simulink model "HT07CombinedPowertrainThermalModel"  (R2022b)
settings: Solver=VariableStepAuto  StartTime=0.0  StopTime=timeEnd  RelTol=1e-4
values from neighbouring files (symbols this model uses):
  Tamb = 26    [HT07CombinedPowertrainThermalSetupExperimental.m]
undefined symbols (not defined in the file or in its folder): AH, convectionArea, DiscIntNeverNeededParam, radiator, SOC0, startTempC, tabResis
libraries: fl_lib x161, nesl_utility x40, SimscapeFluids_lib x16, ee_lib x2
(part 1 of 5)
settings Model: Creator=erc  LastModifiedBy=David
settings SolverCC: MaxConsecutiveMinStep=10
settings DebuggingCC: UnconnectedInputMsg=warning  UnconnectedOutputMsg=warning  UnconnectedLineMsg=warning
settings ModelReferenceCC: EnableRefExpFcnMdlSchedulingChecks=on
settings RTWCC: DLArmComputeVersion=19.05

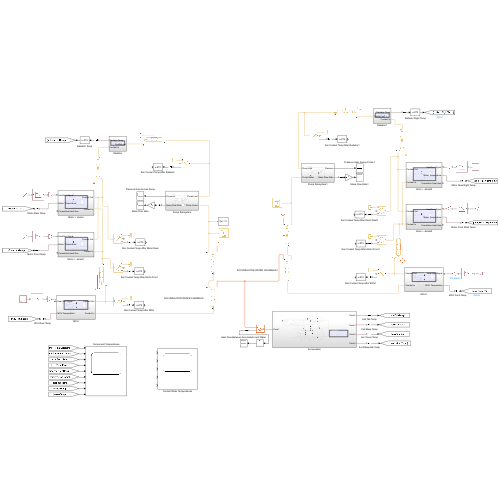
[thumbnail: Simulink's stored preview of the top-level diagram]
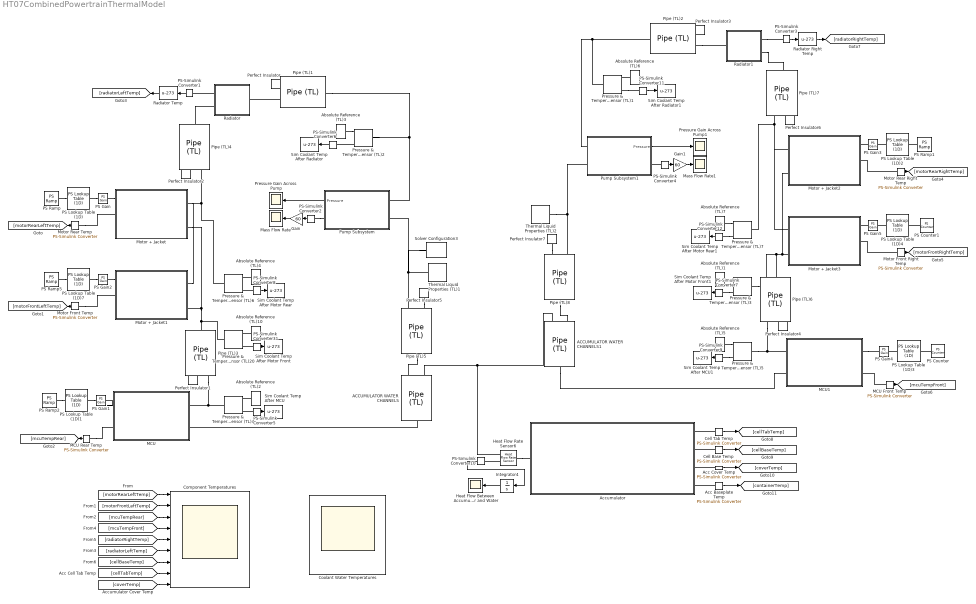
== system HT07CombinedPowertrainThermalModel ==
  ACCUMULATOR WATER CHANNELS : SimscapeFluids_lib/Thermal Liquid/Pipes & Fittings/Pipe (TL)  dynamic_compressibility=simscape.enum.onoff.off  inertia=simscape.enum.onoff.off  num_segments=1  pipe_length=accChannelLength m  area=accChannelFlowArea m^2  wall_spec=fluids.thermal_liquid.pipes_fittings.enum.wall_spec.rigid  Dh=accChannelHydraulicDiameter m  wall_compliance=1.2e-6 m/MPa  wall_time_constant=0.01 s  elevation_spec=foundation.enum.constant_variable.constant  elevation_gain=0 m  g=9.81 m/s^2  pressure_loss_spec=fluids.thermal_liquid.pipes_fittings.enum.PressureLossSpec.Haaland  local_pressure_loss_spec=fluids.thermal_liquid.pipes_fittings.enum.LocalLossSpec.AggregateLength  length_add=0 m  loss_coefficient=0.1  roughness=accChannelAbsoluteRoughness m  Re_friction_TLU=[400, 1000, 1500, 3000, 4000, 6000, 10000, 20000, 40000, 60000, 100000, 100000000]  friction_factor_TLU=[.264, .112, .071, .0417, .0387, .0268, .025, .0232, .0226, .022, .0214, .0214]  shape_factor=64  Re_lam=2000  Re_tur=4000  mdot_nominal=7 kg/min  p_diff_nominal=0.6 bar  mdot_threshold=1e-6 kg/s  heat_transfer_spec=fluids.thermal_liquid.pipes_fittings.enum.HeatTransferSpec.DittusBoelter  mdot_nominal_heat=[.1, 1] kg/s  T_in_nominal=[293.15, 293.15] K  T_out_nominal=[300, 300] K  p_in_nominal_heat=[.101325, .101325] MPa  T_wall_nominal=[303.15, 303.15] K  a_coeff=dittusBoelterAadjAccChannel  b_Re_power=0.8  c_Pr_power=0.4  Nu_lam=3.66  Re_Colburn_TLU=[100, 150, 1000]  Colburn_factor_TLU=[.019, .013, .002]  Re_Nu_TLU=[100, 150, 1000]  Pr_Nu_TLU=[1, 10]  Nu_TLU=[3.72, 4.21; 3.75, 4.44; 4.21, 7.15]  T0_vec=Tamb degC  p0_vec=0.101325 MPa  mdot0=0.1 kg/s
  ACCUMULATOR WATER CHANNELS1 : SimscapeFluids_lib/Thermal Liquid/Pipes & Fittings/Pipe (TL)  dynamic_compressibility=simscape.enum.onoff.off  inertia=simscape.enum.onoff.off  num_segments=1  pipe_length=accChannelLength m  area=accChannelFlowArea m^2  wall_spec=fluids.thermal_liquid.pipes_fittings.enum.wall_spec.rigid  Dh=accChannelHydraulicDiameter m  wall_compliance=1.2e-6 m/MPa  wall_time_constant=0.01 s  elevation_spec=foundation.enum.constant_variable.constant  elevation_gain=0 m  g=9.81 m/s^2  pressure_loss_spec=fluids.thermal_liquid.pipes_fittings.enum.PressureLossSpec.Haaland  local_pressure_loss_spec=fluids.thermal_liquid.pipes_fittings.enum.LocalLossSpec.AggregateLength  length_add=0 m  loss_coefficient=0.1  roughness=accChannelAbsoluteRoughness m  Re_friction_TLU=[400, 1000, 1500, 3000, 4000, 6000, 10000, 20000, 40000, 60000, 100000, 100000000]  friction_factor_TLU=[.264, .112, .071, .0417, .0387, .0268, .025, .0232, .0226, .022, .0214, .0214]  shape_factor=64  Re_lam=2000  Re_tur=4000  mdot_nominal=7 kg/min  p_diff_nominal=0.6 bar  mdot_threshold=1e-6 kg/s  heat_transfer_spec=fluids.thermal_liquid.pipes_fittings.enum.HeatTransferSpec.DittusBoelter  mdot_nominal_heat=[.1, 1] kg/s  T_in_nominal=[293.15, 293.15] K  T_out_nominal=[300, 300] K  p_in_nominal_heat=[.101325, .101325] MPa  T_wall_nominal=[303.15, 303.15] K  a_coeff=dittusBoelterAadjAccChannel  b_Re_power=0.8  c_Pr_power=0.4  Nu_lam=3.66  Re_Colburn_TLU=[100, 150, 1000]  Colburn_factor_TLU=[.019, .013, .002]  Re_Nu_TLU=[100, 150, 1000]  Pr_Nu_TLU=[1, 10]  Nu_TLU=[3.72, 4.21; 3.75, 4.44; 4.21, 7.15]  T0_vec=Tamb degC  p0_vec=0.101325 MPa  mdot0=0.1 kg/s
  Absolute Reference (TL){1..7,10} (8 alike) : fl_lib/Thermal Liquid/Elements/Absolute Reference (TL)
  Acc Baseplate Temp : nesl_utility/PS-Simulink Converter  PhysicalDomain=network_engine_domain  SubClassName=ps_output  LeftPortType=input  RightPortType=output  PseudoPeriodic=off  Frequencies=[]  VectorFormat=inherit  Unit=inherit  AffineConversion=off
  Acc Cover Temp : nesl_utility/PS-Simulink Converter  PhysicalDomain=network_engine_domain  SubClassName=ps_output  LeftPortType=input  RightPortType=output  PseudoPeriodic=off  Frequencies=[]  VectorFormat=inherit  Unit=inherit  AffineConversion=off
  Accumulator : Subsystem
  Cell Base Temp : nesl_utility/PS-Simulink Converter  PhysicalDomain=network_engine_domain  SubClassName=ps_output  LeftPortType=input  RightPortType=output  PseudoPeriodic=off  Frequencies=[]  VectorFormat=inherit  Unit=inherit  AffineConversion=off
  Cell Tab Temp : nesl_utility/PS-Simulink Converter  PhysicalDomain=network_engine_domain  SubClassName=ps_output  LeftPortType=input  RightPortType=output  PseudoPeriodic=off  Frequencies=[]  VectorFormat=inherit  Unit=inherit  AffineConversion=off
  Component Temperatures : Scope  NumInputPorts=9
  Coolant Water Temperatures : Scope  NumInputPorts=5
  Gain : Gain  Gain=60
  Gain1 : Gain  Gain=60
  Heat Flow Between Accumulator and Water : Scope
  Heat Flow Rate Sensor6 : fl_lib/Thermal/Thermal Sensors/Heat Flow Rate Sensor
  Integrator4 : Integrator
  MCU : Subsystem
  MCU Front Temp : nesl_utility/PS-Simulink Converter  PhysicalDomain=network_engine_domain  SubClassName=ps_output  LeftPortType=input  RightPortType=output  PseudoPeriodic=off  Frequencies=[]  VectorFormat=inherit  Unit=inherit  AffineConversion=off
  MCU Rear Temp : nesl_utility/PS-Simulink Converter  PhysicalDomain=network_engine_domain  SubClassName=ps_output  LeftPortType=input  RightPortType=output  PseudoPeriodic=off  Frequencies=[]  VectorFormat=inherit  Unit=inherit  AffineConversion=off
  MCU1 : Subsystem
  Mass Flow Rate : Scope
  Mass Flow Rate1 : Scope
  Motor + Jacket : Subsystem
  Motor + Jacket1 : Subsystem
  Motor + Jacket2 : Subsystem
  Motor + Jacket3 : Subsystem
  Motor Front Right Temp : nesl_utility/PS-Simulink Converter  PhysicalDomain=network_engine_domain  SubClassName=ps_output  LeftPortType=input  RightPortType=output  PseudoPeriodic=off  Frequencies=[]  VectorFormat=inherit  Unit=inherit  AffineConversion=off
  Motor Front Temp : nesl_utility/PS-Simulink Converter  PhysicalDomain=network_engine_domain  SubClassName=ps_output  LeftPortType=input  RightPortType=output  PseudoPeriodic=off  Frequencies=[]  VectorFormat=inherit  Unit=inherit  AffineConversion=off
  Motor Rear Right Temp : nesl_utility/PS-Simulink Converter  PhysicalDomain=network_engine_domain  SubClassName=ps_output  LeftPortType=input  RightPortType=output  PseudoPeriodic=off  Frequencies=[]  VectorFormat=inherit  Unit=inherit  AffineConversion=off
  Motor Rear Temp : nesl_utility/PS-Simulink Converter  PhysicalDomain=network_engine_domain  SubClassName=ps_output  LeftPortType=input  RightPortType=output  PseudoPeriodic=off  Frequencies=[]  VectorFormat=inherit  Unit=inherit  AffineConversion=off
  PS Counter : fl_lib/Physical Signals/Sources/PS Counter  sample_time=1 s  init_val=0  reset_val=0  max_val=intmax
      settings: InternalSimscapePortConfiguration="{\"Bottom\":[],\"Left\":[],\"Right\":[{\"id\":\"Y\",\"label\":\"Y\",\"type\":\"output\"}],\"Top\":[]}"
  PS Counter1 : fl_lib/Physical Signals/Sources/PS Counter  sample_time=1 s  init_val=0  reset_val=0  max_val=intmax
      settings: InternalSimscapePortConfiguration="{\"Bottom\":[],\"Left\":[],\"Right\":[{\"id\":\"Y\",\"label\":\"Y\",\"type\":\"output\"}],\"Top\":[]}"
  PS Gain{,2..3,5} (4 alike) : fl_lib/Physical Signals/Functions/PS Gain  gain=1
  PS Gain1 : fl_lib/Physical Signals/Functions/PS Gain  gain=2
  PS Gain4 : fl_lib/Physical Signals/Functions/PS Gain  gain=2
  PS Lookup Table (1D) : fl_lib/Physical Signals/Lookup Tables/PS Lookup Table (1D)  x=time  f=motorRearHeatGen J/s  interp_method=simscape.enum.interpolation.linear  extrap_method=simscape.enum.extrapolation.nearest
  PS Lookup Table (1D)1 : fl_lib/Physical Signals/Lookup Tables/PS Lookup Table (1D)  x=time  f=mcuHeatGen J/s  interp_method=simscape.enum.interpolation.linear  extrap_method=simscape.enum.extrapolation.nearest
  PS Lookup Table (1D)2 : fl_lib/Physical Signals/Lookup Tables/PS Lookup Table (1D)  x=time  f=motorRearHeatGen J/s  interp_method=simscape.enum.interpolation.linear  extrap_method=simscape.enum.extrapolation.nearest
  PS Lookup Table (1D)3 : fl_lib/Physical Signals/Lookup Tables/PS Lookup Table (1D)  x=time  f=mcuHeatGen J/s  interp_method=simscape.enum.interpolation.linear  extrap_method=simscape.enum.extrapolation.nearest
  PS Lookup Table (1D)4 : fl_lib/Physical Signals/Lookup Tables/PS Lookup Table (1D)  x=time  f=motorFrontHeatGen J/s  interp_method=simscape.enum.interpolation.linear  extrap_method=simscape.enum.extrapolation.nearest
  PS Lookup Table (1D)7 : fl_lib/Physical Signals/Lookup Tables/PS Lookup Table (1D)  x=time  f=motorFrontHeatGen J/s  interp_method=simscape.enum.interpolation.linear  extrap_method=simscape.enum.extrapolation.nearest
  PS Ramp{,1..2,5} (4 alike) : fl_lib/Physical Signals/Sources/PS Ramp  slope=1 1/s  start_time=0 s  initial_output=0
  PS-Simulink Converter{1,3,5..9,11..12,31} (10 alike) : nesl_utility/PS-Simulink Converter  PhysicalDomain=network_engine_domain  SubClassName=ps_output  LeftPortType=input  RightPortType=output  PseudoPeriodic=off  Frequencies=[]  VectorFormat=inherit  Unit=inherit  AffineConversion=off
  PS-Simulink Converter10 : nesl_utility/PS-Simulink Converter  PhysicalDomain=network_engine_domain  SubClassName=ps_output  LeftPortType=input  RightPortType=output  PseudoPeriodic=off  Frequencies=[]  VectorFormat=1-D array  Unit=inherit  AffineConversion=off
  PS-Simulink Converter2 : nesl_utility/PS-Simulink Converter  PhysicalDomain=network_engine_domain  SubClassName=ps_output  LeftPortType=input  RightPortType=output  PseudoPeriodic=off  Frequencies=[]  VectorFormat=1-D array  Unit=inherit  AffineConversion=off
  PS-Simulink Converter4 : nesl_utility/PS-Simulink Converter  PhysicalDomain=network_engine_domain  SubClassName=ps_output  LeftPortType=input  RightPortType=output  PseudoPeriodic=off  Frequencies=[]  VectorFormat=1-D array  Unit=inherit  AffineConversion=off
  Perfect Insulator{,1..7} (8 alike) : fl_lib/Thermal/Thermal Elements/Perfect Insulator  T_specify=off  T_priority=None  T=0 K  T_nominal_specify=off  T_nominal_unit=K  T_nominal_value=1
  Pipe (TL)1 : fl_lib/Thermal Liquid/Elements/Pipe (TL)  length=tubeLengthRadiatorToPump m  area=A m^2  Dh=d m  length_add=0 m  roughness=tubeRoughness m  Re_lam=2000  Re_tur=4000  shape_factor=64  Nu_lam=3.66  dynamic_compressibility=simscape.enum.onoff.off  inertia=simscape.enum.onoff.off  p0=0.101325 MPa  T0=Tamb degC  mdot0=0 kg/s
  Pipe (TL)2 : fl_lib/Thermal Liquid/Elements/Pipe (TL)  length=tubeLengthRadiatorToPump m  area=A m^2  Dh=d m  length_add=0 m  roughness=tubeRoughness m  Re_lam=2000  Re_tur=4000  shape_factor=64  Nu_lam=3.66  dynamic_compressibility=simscape.enum.onoff.off  inertia=simscape.enum.onoff.off  p0=0.101325 MPa  T0=Tamb degC  mdot0=0 kg/s
  Pipe (TL)3 : fl_lib/Thermal Liquid/Elements/Pipe (TL)  length=tubeLengthMCUToMotor m  area=A m^2  Dh=d m  length_add=leqMCUToMotor m  roughness=tubeRoughness m  Re_lam=2000  Re_tur=4000  shape_factor=64  Nu_lam=3.66  dynamic_compressibility=simscape.enum.onoff.off  inertia=simscape.enum.onoff.off  p0=0.101325 MPa  T0=Tamb degC  mdot0=0 kg/s
  Pipe (TL)4 : fl_lib/Thermal Liquid/Elements/Pipe (TL)  length=tubeLengthMotorToRadiator m  area=A m^2  Dh=d m  length_add=leqMotorToRadiator m  roughness=tubeRoughness m  Re_lam=2000  Re_tur=4000  shape_factor=64  Nu_lam=3.66  dynamic_compressibility=simscape.enum.onoff.off  inertia=simscape.enum.onoff.off  p0=0.101325 MPa  T0=Tamb degC  mdot0=0 kg/s
  Pipe (TL)5 : fl_lib/Thermal Liquid/Elements/Pipe (TL)  length=tubeLengthPumpToMCU m  area=A m^2  Dh=d m  length_add=leqMCUToMotor m  roughness=tubeRoughness m  Re_lam=2000  Re_tur=4000  shape_factor=64  Nu_lam=3.66  dynamic_compressibility=simscape.enum.onoff.off  inertia=simscape.enum.onoff.off  p0=0.101325 MPa  T0=Tamb degC  mdot0=0 kg/s
  Pipe (TL)6 : fl_lib/Thermal Liquid/Elements/Pipe (TL)  length=tubeLengthMCUToMotor m  area=A m^2  Dh=d m  length_add=leqMCUToMotor m  roughness=tubeRoughness m  Re_lam=2000  Re_tur=4000  shape_factor=64  Nu_lam=3.66  dynamic_compressibility=simscape.enum.onoff.off  inertia=simscape.enum.onoff.off  p0=0.101325 MPa  T0=Tamb degC  mdot0=0 kg/s
  Pipe (TL)7 : fl_lib/Thermal Liquid/Elements/Pipe (TL)  length=tubeLengthMotorToRadiator m  area=A m^2  Dh=d m  length_add=leqMotorToRadiator m  roughness=tubeRoughness m  Re_lam=2000  Re_tur=4000  shape_factor=64  Nu_lam=3.66  dynamic_compressibility=simscape.enum.onoff.off  inertia=simscape.enum.onoff.off  p0=0.101325 MPa  T0=Tamb degC  mdot0=0 kg/s
  Pipe (TL)8 : fl_lib/Thermal Liquid/Elements/Pipe (TL)  length=tubeLengthPumpToMCU m  area=A m^2  Dh=d m  length_add=leqMCUToMotor m  roughness=tubeRoughness m  Re_lam=2000  Re_tur=4000  shape_factor=64  Nu_lam=3.66  dynamic_compressibility=simscape.enum.onoff.off  inertia=simscape.enum.onoff.off  p0=0.101325 MPa  T0=Tamb degC  mdot0=0 kg/s
  Pressure & Temperature Sensor (TL){1..7,20} (8 alike) : fl_lib/Thermal Liquid/Sensors/Pressure & Temperature Sensor (TL)
      settings: InternalSimscapePortConfiguration="{\"Bottom\":[],\"Left\":[{\"id\":\"A\",\"label\":\"A\",\"type\":\"foundation.thermal_liquid.thermal_liquid\"}],\"Right\":[{\"id\":\"B\",\"label\":\"B\",\"type\":\"foundation.thermal_liquid.thermal_liquid\"},{\"id\":\"P\",\"label\":\"P\",\"type\":\"output\"},{\"id\":\"T\",\"label\":\"T\",\"type\":\"output\"}],\"Top\":[]}"
  Pressure Gain Across Pump : Scope
  Pressure Gain Across Pump1 : Scope
  Pump Subsystem : Subsystem
  Pump Subsystem1 : Subsystem
  Radiator : Subsystem
  Radiator Right Temp : Bias  Bias=-273  SaturateOnIntegerOverflow=off
  Radiator Temp : Bias  Bias=-273  SaturateOnIntegerOverflow=off
  Radiator1 : Subsystem
  Sim Coolant Temp After MCU : Bias  Bias=-273  SaturateOnIntegerOverflow=off
  Sim Coolant Temp After MCU1 : Bias  Bias=-273  SaturateOnIntegerOverflow=off
  Sim Coolant Temp After Motor Front : Bias  Bias=-273  SaturateOnIntegerOverflow=off
  Sim Coolant Temp After Motor Front1 : Bias  Bias=-273  SaturateOnIntegerOverflow=off
  Sim Coolant Temp After Motor Rear : Bias  Bias=-273  SaturateOnIntegerOverflow=off
  Sim Coolant Temp After Motor Rear1 : Bias  Bias=-273  SaturateOnIntegerOverflow=off
  Sim Coolant Temp After Radiator : Bias  Bias=-273  SaturateOnIntegerOverflow=off
  Sim Coolant Temp After Radiator1 : Bias  Bias=-273  SaturateOnIntegerOverflow=off
  Solver Configuration3 : nesl_utility/Solver Configuration  PhysicalDomain=network_engine_domain  SubClassName=solver  LeftPortType=input  RightPortType=generic  Tones=[]  Harmonics=[]  SimulateNoise=off  Profile=off  UseLocalSampling=off  EnableSwitchedLinearOptims=on  FrequencyDomain=off  UseCCode=off  RelTol=0.001  AbsTol=1e-06  MinStep=1e-09  ToWorkspace=off  RevertToSquareIcSolve=off  NumHomotopyIterations=100  PhasorMode=off  PhasorModeNumHarmonics=1  ConsistencySolver=NEWTON_FTOL  IndexReductionMethod=DerivativeReplacement  DoDC=on  ResidualTolerance=1e-08  ConsistencyTolSource=GLOBAL  ConsistencyAbsTol=0.001  ConsistencyRelTol=0.001  ConsistencyTolFactor=0.001  UseLocalSolver=off  LocalSolverChoice=NE_BACKWARD_EULER_ADVANCER  ResolveIndetEquations=on  FunctionEvalNumThread=1  LocalSolverSampleTime=0.001  DoFixedCost=off  MaxNonlinIter=3  MaxModeIter=2  ComputeImpulses=off  ImpulseIterations=2  LinearAlgebra=auto  LinearAlgebraNumThread=0  EquationFormulation=NE_TIME_EF  DelaysMemoryBudget=1024  AutomaticFiltering=on  FilteringTimeConstant=0.001  PartitionStorageMethod=AS_NEEDED  PartitionMemoryBudget=1024  PartitionMethod=ROBUST
  Thermal Liquid Properties (TL)1 : SimscapeFluids_lib/Thermal Liquid/Utilities/Thermal Liquid Properties (TL)  fluid_list=fluids.thermal_liquid.utilities.enum.thermal_liquid_fluid_list.water  concentration_param_EG=fluids.thermal_liquid.utilities.enum.thermal_liquid_concentration.volume_fraction  concentration_param_PG=fluids.thermal_liquid.utilities.enum.thermal_liquid_concentration.volume_fraction  c_mass_SW=3.5e-3  c_mass_EG=0.1  c_mass_PG=0.1  c_mass_GL=0.1  c_vol_EG=0.1  c_vol_PG=0.1  beta_const_EG=2.1791 GPa  beta_const_PG=2.1791 GPa  beta_const_GL=2.1791 GPa  p_min_EG=0.01 MPa  p_min_PG=0.01 MPa  p_min_GL=0.01 MPa  p_max_EG=50 MPa  p_max_PG=50 MPa  p_max_GL=50 MPa  p_atm=0.101325 MPa
  Thermal Liquid Properties (TL)2 : SimscapeFluids_lib/Thermal Liquid/Utilities/Thermal Liquid Properties (TL)  fluid_list=fluids.thermal_liquid.utilities.enum.thermal_liquid_fluid_list.water  concentration_param_EG=fluids.thermal_liquid.utilities.enum.thermal_liquid_concentration.volume_fraction  concentration_param_PG=fluids.thermal_liquid.utilities.enum.thermal_liquid_concentration.volume_fraction  c_mass_SW=3.5e-3  c_mass_EG=0.1  c_mass_PG=0.1  c_mass_GL=0.1  c_vol_EG=0.1  c_vol_PG=0.1  beta_const_EG=2.1791 GPa  beta_const_PG=2.1791 GPa  beta_const_GL=2.1791 GPa  p_min_EG=0.01 MPa  p_min_PG=0.01 MPa  p_min_GL=0.01 MPa  p_max_EG=50 MPa  p_max_PG=50 MPa  p_max_GL=50 MPa  p_atm=0.101325 MPa
  wires:
  PS-Simulink Converter6/1 -> Sim Coolant Temp After Radiator/1
  PS-Simulink Converter5/1 -> Sim Coolant Temp After MCU/1
  PS-Simulink Converter8/1 -> Sim Coolant Temp After Motor Rear/1
  PS-Simulink Converter31/1 -> Sim Coolant Temp After Motor Front/1
  Integrator4/1 -> Heat Flow Between Accumulator and Water/1
  PS-Simulink Converter10/1 -> Integrator4/1
  Motor Rear Temp/1 -> [motorRearLeftTemp]
  [motorRearLeftTemp] -> Component Temperatures/1
  Motor Front Temp/1 -> [motorFrontLeftTemp]
  [motorFrontLeftTemp] -> Component Temperatures/2
  MCU Rear Temp/1 -> [mcuTempRear]
  [mcuTempRear] -> Component Temperatures/3
  Pump Subsystem/1(Pressure) -> Pressure Gain Across Pump/1
  PS-Simulink Converter1/1 -> Radiator Temp/1
  [radiatorLeftTemp] -> Component Temperatures/6
  PS-Simulink Converter2/1 -> Gain/1
  Gain/1 -> Mass Flow Rate/1
  Radiator Temp/1 -> [radiatorLeftTemp]
  Motor Rear Right Temp/1 -> [motorRearRightTemp]
  PS-Simulink Converter7/1 -> Sim Coolant Temp After Motor Front1/1
  Motor Front Right Temp/1 -> [motorFrontRightTemp]
  PS-Simulink Converter9/1 -> Sim Coolant Temp After MCU1/1
  Pump Subsystem1/1(Pressure) -> Pressure Gain Across Pump1/1
  PS-Simulink Converter12/1 -> Sim Coolant Temp After Motor Rear1/1
  Gain1/1 -> Mass Flow Rate1/1
  PS-Simulink Converter4/1 -> Gain1/1
  Radiator Right Temp/1 -> [radiatorRightTemp]
  PS-Simulink Converter11/1 -> Sim Coolant Temp After Radiator1/1
  PS-Simulink Converter3/1 -> Radiator Right Temp/1
  MCU Front Temp/1 -> [mcuTempFront]
  [mcuTempFront] -> Component Temperatures/4
  Cell Tab Temp/1 -> [cellTabTemp]
  Cell Base Temp/1 -> [cellBaseTemp]
  Acc Cover Temp/1 -> [coverTemp]
  Acc Baseplate Temp/1 -> [containerTemp]
  [radiatorRightTemp] -> Component Temperatures/5
  [cellBaseTemp] -> Component Temperatures/7
  [coverTemp] -> Component Temperatures/9
  [cellTabTemp] -> Component Temperatures/8
  connections:
  PS Lookup Table (1D)1/RConn1 -- PS Gain1/LConn1
  PS Ramp2/RConn1 -- PS Lookup Table (1D)1/LConn1
  Perfect Insulator/LConn1 -- Pipe (TL)1/LConn2
  Thermal Liquid Properties (TL)1/RConn1 -- Solver Configuration3/RConn1 -- Pump Subsystem/LConn2 -- Pipe (TL)5/LConn1
  Absolute Reference (TL)3/LConn1 -- Pressure & Temperature Sensor (TL)2/RConn1
  Pressure & Temperature Sensor (TL)2/RConn3 -- PS-Simulink Converter6/LConn1
  Perfect Insulator1/LConn1 -- Pipe (TL)3/LConn2
  Pipe (TL)4/LConn2 -- Perfect Insulator2/LConn1
  Perfect Insulator5/LConn1 -- Pipe (TL)5/LConn2
  Pressure & Temperature Sensor (TL)6/LConn1 -- Motor + Jacket1/LConn1 -- Motor + Jacket/LConn1 -- Pipe (TL)4/LConn1
  ACCUMULATOR WATER CHANNELS/RConn1 -- MCU/RConn2
  Pipe (TL)3/LConn1 -- MCU/RConn1 -- Pressure & Temperature Sensor (TL)4/LConn1
  Absolute Reference (TL)2/LConn1 -- Pressure & Temperature Sensor (TL)4/RConn1
  PS-Simulink Converter5/LConn1 -- Pressure & Temperature Sensor (TL)4/RConn3
  Absolute Reference (TL)4/LConn1 -- Pressure & Temperature Sensor (TL)6/RConn1
  PS-Simulink Converter8/LConn1 -- Pressure & Temperature Sensor (TL)6/RConn3
  PS Lookup Table (1D)/RConn1 -- PS Gain/LConn1
  PS Ramp/RConn1 -- PS Lookup Table (1D)/LConn1
  PS Lookup Table (1D)7/RConn1 -- PS Gain2/LConn1
  PS Ramp5/RConn1 -- PS Lookup Table (1D)7/LConn1
  PS-Simulink Converter31/LConn1 -- Pressure & Temperature Sensor (TL)20/RConn3
  Absolute Reference (TL)10/LConn1 -- Pressure & Temperature Sensor (TL)20/RConn1
  Pipe (TL)5/RConn1 -- ACCUMULATOR WATER CHANNELS/LConn1
  Heat Flow Rate Sensor6/RConn1 -- PS-Simulink Converter10/LConn1
  ACCUMULATOR WATER CHANNELS/LConn2 -- ACCUMULATOR WATER CHANNELS1/LConn2 -- Heat Flow Rate Sensor6/RConn2
  Pressure & Temperature Sensor (TL)20/LConn1 -- Motor + Jacket/LConn2 -- Motor + Jacket1/LConn2 -- Pipe (TL)3/RConn1
  Pipe (TL)1/LConn1 -- Radiator/LConn1
  Radiator/RConn2 -- Pipe (TL)4/RConn1
  PS Gain/RConn1 -- Motor + Jacket/RConn1
  Motor Rear Temp/LConn1 -- Motor + Jacket/RConn2
  PS Gain2/RConn1 -- Motor + Jacket1/RConn1
  Motor Front Temp/LConn1 -- Motor + Jacket1/RConn2
  MCU/LConn1 -- PS Gain1/RConn1
  MCU Rear Temp/LConn1 -- MCU/LConn2
  Pressure & Temperature Sensor (TL)2/LConn1 -- Pump Subsystem/LConn1 -- Pipe (TL)1/RConn1
  Radiator/RConn1 -- PS-Simulink Converter1/LConn1
  PS-Simulink Converter2/LConn1 -- Pump Subsystem/RConn1
  Heat Flow Rate Sensor6/LConn1 -- Accumulator/LConn1
  Pressure & Temperature Sensor (TL)3/LConn1 -- Pipe (TL)6/RConn1 -- Motor + Jacket2/LConn2 -- Motor + Jacket3/LConn2
  Pipe (TL)6/LConn1 -- Pressure & Temperature Sensor (TL)5/LConn1 -- MCU1/RConn1
  Thermal Liquid Properties (TL)2/RConn1 -- Pipe (TL)8/LConn1 -- Pump Subsystem1/LConn2
  Pressure & Temperature Sensor (TL)7/LConn1 -- Motor + Jacket3/LConn1 -- Motor + Jacket2/LConn1 -- Pipe (TL)7/LConn1
  Pressure & Temperature Sensor (TL)1/LConn1 -- Pipe (TL)2/RConn1 -- Pump Subsystem1/LConn1
  PS Counter1/RConn1 -- PS Lookup Table (1D)4/LConn1
  Perfect Insulator7/LConn1 -- Pipe (TL)8/LConn2
  Radiator1/RConn2 -- Pipe (TL)7/RConn1
  PS-Simulink Converter7/LConn1 -- Pressure & Temperature Sensor (TL)3/RConn3
  Absolute Reference (TL)1/LConn1 -- Pressure & Temperature Sensor (TL)3/RConn1
  MCU1/LConn1 -- PS Gain4/RConn1
  Pipe (TL)8/RConn1 -- ACCUMULATOR WATER CHANNELS1/LConn1
  Absolute Reference (TL)5/LConn1 -- Pressure & Temperature Sensor (TL)5/RConn1
  PS Lookup Table (1D)4/RConn1 -- PS Gain5/LConn1
  Pipe (TL)2/LConn1 -- Radiator1/LConn1
  PS-Simulink Converter4/LConn1 -- Pump Subsystem1/RConn1
  PS-Simulink Converter9/LConn1 -- Pressure & Temperature Sensor (TL)5/RConn3
  Motor Front Right Temp/LConn1 -- Motor + Jacket3/RConn2
  PS Ramp1/RConn1 -- PS Lookup Table (1D)2/LConn1
  MCU Front Temp/LConn1 -- MCU1/LConn2
  Radiator1/RConn1 -- PS-Simulink Converter3/LConn1
  ACCUMULATOR WATER CHANNELS1/RConn1 -- MCU1/RConn2
  Absolute Reference (TL)7/LConn1 -- Pressure & Temperature Sensor (TL)7/RConn1
  PS Lookup Table (1D)3/RConn1 -- PS Gain4/LConn1
  Perfect Insulator3/LConn1 -- Pipe (TL)2/LConn2
  PS Gain3/RConn1 -- Motor + Jacket2/RConn1
  PS Lookup Table (1D)2/RConn1 -- PS Gain3/LConn1
  Absolute Reference (TL)6/LConn1 -- Pressure & Temperature Sensor (TL)1/RConn1
  Pressure & Temperature Sensor (TL)1/RConn3 -- PS-Simulink Converter11/LConn1
  Perfect Insulator4/LConn1 -- Pipe (TL)6/LConn2
  PS-Simulink Converter12/LConn1 -- Pressure & Temperature Sensor (TL)7/RConn3
  PS Gain5/RConn1 -- Motor + Jacket3/RConn1
  Motor Rear Right Temp/LConn1 -- Motor + Jacket2/RConn2
  Pipe (TL)7/LConn2 -- Perfect Insulator6/LConn1
  PS Counter/RConn1 -- PS Lookup Table (1D)3/LConn1
  Cell Tab Temp/LConn1 -- Accumulator/RConn1
  Cell Base Temp/LConn1 -- Accumulator/RConn2
  Acc Cover Temp/LConn1 -- Accumulator/RConn3
  Acc Baseplate Temp/LConn1 -- Accumulator/RConn4

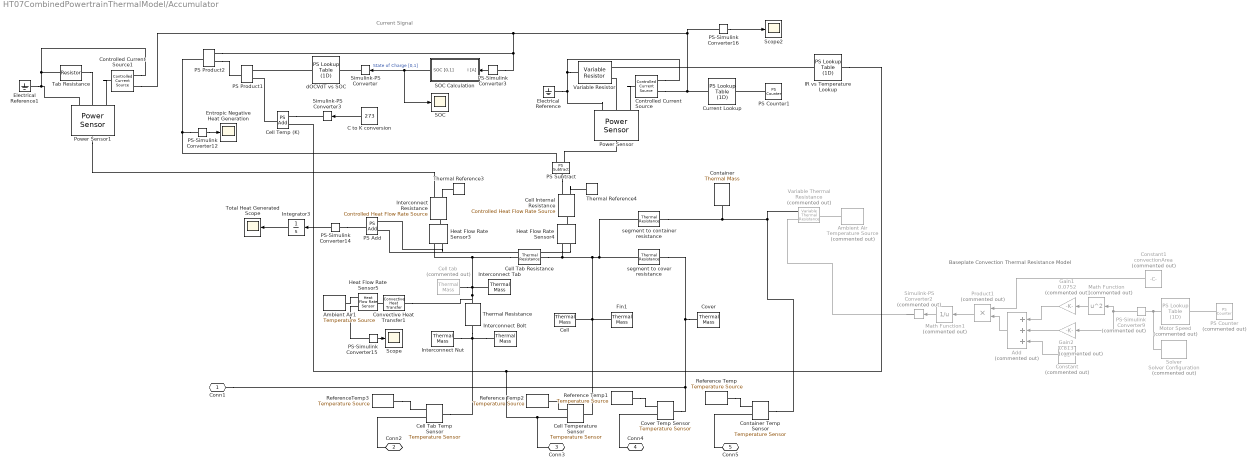
== system HT07CombinedPowertrainThermalModel/Accumulator ==
  note: Baseplate Convection Thermal Resistance Model
  note: Current Signal
  " Fin1" : fl_lib/Thermal/Thermal Elements/Thermal Mass  mass=mFin kg  sp_heat=cAl J/kg/K  num_ports=foundation.enum.numPorts2.one  T_specify=on  T_priority=High  T=startTempC degC  T_nominal_specify=off  T_nominal_unit=K  T_nominal_value=1  Q_specify=off  Q_priority=None  Q=0 W  Q_nominal_specify=off  Q_nominal_unit=W  Q_nominal_value=1
  Add : Sum  Commented=on  Inputs=+++
  Ambient Air : fl_lib/Thermal/Thermal Sources/Temperature Source  Commented=on  temperature=startTempC degC
  Ambient Air1 : fl_lib/Thermal/Thermal Sources/Temperature Source  temperature=startTempC degC
  C to K conversion : Constant  Value=273
  "Cell " : fl_lib/Thermal/Thermal Elements/Thermal Mass  mass=mCell kg  sp_heat=cCell J/kg/K  num_ports=foundation.enum.numPorts2.one  T_specify=on  T_priority=High  T=startTempC degC  T_nominal_specify=off  T_nominal_unit=K  T_nominal_value=1  Q_specify=off  Q_priority=None  Q=0 W  Q_nominal_specify=off  Q_nominal_unit=W  Q_nominal_value=1
  Cell Internal Resistance : fl_lib/Thermal/Thermal Sources/Controlled Heat Flow Rate Source
  Cell Tab Resistance : fl_lib/Thermal/Thermal Elements/Thermal Resistance  resistance=R_tc K/W  T_specify=off  T_priority=None  T=0 K  T_nominal_specify=off  T_nominal_unit=K  T_nominal_value=1  Q_specify=off  Q_priority=None  Q=0 W  Q_nominal_specify=off  Q_nominal_unit=W  Q_nominal_value=1
  Cell Tab Temp Sensor : fl_lib/Thermal/Thermal Sensors/Temperature Sensor
  Cell Temp (K) : fl_lib/Physical Signals/Functions/PS Add
  Cell Temperature Sensor : fl_lib/Thermal/Thermal Sensors/Temperature Sensor
  Cell tab : fl_lib/Thermal/Thermal Elements/Thermal Mass  Commented=on  mass=cellTabThermalMass kg  sp_heat=cCu J/kg/K  num_ports=foundation.enum.numPorts2.one  T_specify=on  T_priority=High  T=startTempC degC  T_nominal_specify=off  T_nominal_unit=K  T_nominal_value=1  Q_specify=off  Q_priority=None  Q=0 W  Q_nominal_specify=off  Q_nominal_unit=W  Q_nominal_value=1
  Constant : Constant  Commented=on  Value=30
  Constant1 : Constant  Commented=on  Value=convectionArea
  Container : fl_lib/Thermal/Thermal Elements/Thermal Mass  mass=mContainerAdj kg  sp_heat=cAl J/kg/K  num_ports=foundation.enum.numPorts2.one  T_specify=on  T_priority=High  T=startTempC degC  T_nominal_specify=off  T_nominal_unit=K  T_nominal_value=1  Q_specify=off  Q_priority=None  Q=0 W  Q_nominal_specify=off  Q_nominal_unit=W  Q_nominal_value=1
  Container Temp Sensor : fl_lib/Thermal/Thermal Sensors/Temperature Sensor
  Controlled Current Source : fl_lib/Electrical/Electrical Sources/Controlled Current Source
  Controlled Current Source1 : fl_lib/Electrical/Electrical Sources/Controlled Current Source
  Convective Heat Transfer1 : fl_lib/Thermal/Thermal Elements/Convective Heat Transfer  thermal_type=foundation.enum.constant_variable.constant  area=tabConvectionArea m^2  heat_tr_coeff=tabConvectionCoefficient W/(m^2*K)  min_heat_tr_coeff=1e-3 W/(K*m^2)  T_specify=off  T_priority=None  T=0 K  T_nominal_specify=off  T_nominal_unit=K  T_nominal_value=1  Q_specify=off  Q_priority=None  Q=0 W  Q_nominal_specify=off  Q_nominal_unit=W  Q_nominal_value=1
  Cover : fl_lib/Thermal/Thermal Elements/Thermal Mass  mass=mCoverAdj kg  sp_heat=cAl J/kg/K  num_ports=foundation.enum.numPorts2.one  T_specify=on  T_priority=High  T=startTempC degC  T_nominal_specify=off  T_nominal_unit=K  T_nominal_value=1  Q_specify=off  Q_priority=None  Q=0 W  Q_nominal_specify=off  Q_nominal_unit=W  Q_nominal_value=1
  Cover Temp Sensor : fl_lib/Thermal/Thermal Sensors/Temperature Sensor
  Current Lookup : fl_lib/Physical Signals/Lookup Tables/PS Lookup Table (1D)  x=time  f=current A  interp_method=simscape.enum.interpolation.linear  extrap_method=simscape.enum.extrapolation.nearest
  Electrical Reference : fl_lib/Electrical/Electrical Elements/Electrical Reference
  Electrical Reference1 : fl_lib/Electrical/Electrical Elements/Electrical Reference
  Entropic Negative Heat Generation : Scope
  Gain1 : Gain  Commented=on  Gain=0.0752
  Gain2 : Gain  Commented=on  Gain=0.813
  Heat Flow Rate Sensor3 : fl_lib/Thermal/Thermal Sensors/Heat Flow Rate Sensor
  Heat Flow Rate Sensor4 : fl_lib/Thermal/Thermal Sensors/Heat Flow Rate Sensor
  Heat Flow Rate Sensor5 : fl_lib/Thermal/Thermal Sensors/Heat Flow Rate Sensor
  IR vs Temperature Lookup : fl_lib/Physical Signals/Lookup Tables/PS Lookup Table (1D)  x=tempVec K  f=IRVec Ohm  interp_method=simscape.enum.interpolation.linear  extrap_method=simscape.enum.extrapolation.nearest
  Integrator3 : Integrator
  Interconnect Bolt : fl_lib/Thermal/Thermal Elements/Thermal Mass  mass=mInterconnectBoltTotal kg  sp_heat=cSt J/kg/K  num_ports=foundation.enum.numPorts2.one  T_specify=on  T_priority=High  T=startTempC degC  T_nominal_specify=off  T_nominal_unit=K  T_nominal_value=1  Q_specify=off  Q_priority=None  Q=0 W  Q_nominal_specify=off  Q_nominal_unit=W  Q_nominal_value=1
  Interconnect Nut : fl_lib/Thermal/Thermal Elements/Thermal Mass  mass=mInterconnectNutTotal kg  sp_heat=cSt J/kg/K  num_ports=foundation.enum.numPorts2.one  T_specify=on  T_priority=High  T=startTempC degC  T_nominal_specify=off  T_nominal_unit=K  T_nominal_value=1  Q_specify=off  Q_priority=None  Q=0 W  Q_nominal_specify=off  Q_nominal_unit=W  Q_nominal_value=1
  Interconnect Resistance : fl_lib/Thermal/Thermal Sources/Controlled Heat Flow Rate Source
  Interconnect Tab : fl_lib/Thermal/Thermal Elements/Thermal Mass  mass=mInterconnect kg  sp_heat=cAl J/kg/K  num_ports=foundation.enum.numPorts2.one  T_specify=on  T_priority=High  T=startTempC degC  T_nominal_specify=off  T_nominal_unit=K  T_nominal_value=1  Q_specify=off  Q_priority=None  Q=0 W  Q_nominal_specify=off  Q_nominal_unit=W  Q_nominal_value=1
  Math Function : Math  Commented=on  Operator=square
  Math Function1 : Math  Commented=on  Operator=reciprocal
  Motor Speed : fl_lib/Physical Signals/Lookup Tables/PS Lookup Table (1D)  Commented=on  x=time  f=velocity  interp_method=simscape.enum.interpolation.linear  extrap_method=simscape.enum.extrapolation.nearest
  PS Add : fl_lib/Physical Signals/Functions/PS Add
  PS Counter : fl_lib/Physical Signals/Sources/PS Counter  Commented=on  sample_time=1 s  init_val=0  reset_val=0  max_val=intmax
      settings: InternalSimscapePortConfiguration="{\"Bottom\":[],\"Left\":[],\"Right\":[{\"id\":\"Y\",\"label\":\"Y\",\"type\":\"output\"}],\"Top\":[]}"
  PS Counter1 : fl_lib/Physical Signals/Sources/PS Counter  sample_time=1 s  init_val=0  reset_val=0  max_val=intmax
      settings: InternalSimscapePortConfiguration="{\"Bottom\":[],\"Left\":[],\"Right\":[{\"id\":\"Y\",\"label\":\"Y\",\"type\":\"output\"}],\"Top\":[]}"
  PS Product1 : fl_lib/Physical Signals/Functions/PS Product
  PS Product2 : fl_lib/Physical Signals/Functions/PS Product
  PS Subtract : fl_lib/Physical Signals/Functions/PS Subtract
  PS-Simulink Converter12 : nesl_utility/PS-Simulink Converter  PhysicalDomain=network_engine_domain  SubClassName=ps_output  LeftPortType=input  RightPortType=output  PseudoPeriodic=off  Frequencies=[]  VectorFormat=1-D array  Unit=inherit  AffineConversion=off
  PS-Simulink Converter14 : nesl_utility/PS-Simulink Converter  PhysicalDomain=network_engine_domain  SubClassName=ps_output  LeftPortType=input  RightPortType=output  PseudoPeriodic=off  Frequencies=[]  VectorFormat=1-D array  Unit=inherit  AffineConversion=off
  PS-Simulink Converter15 : nesl_utility/PS-Simulink Converter  PhysicalDomain=network_engine_domain  SubClassName=ps_output  LeftPortType=input  RightPortType=output  PseudoPeriodic=off  Frequencies=[]  VectorFormat=inherit  Unit=inherit  AffineConversion=off
  PS-Simulink Converter16 : nesl_utility/PS-Simulink Converter  PhysicalDomain=network_engine_domain  SubClassName=ps_output  LeftPortType=input  RightPortType=output  PseudoPeriodic=off  Frequencies=[]  VectorFormat=inherit  Unit=inherit  AffineConversion=off
  PS-Simulink Converter3 : nesl_utility/PS-Simulink Converter  PhysicalDomain=network_engine_domain  SubClassName=ps_output  LeftPortType=input  RightPortType=output  PseudoPeriodic=off  Frequencies=[]  VectorFormat=1-D array  Unit=inherit  AffineConversion=off
  PS-Simulink Converter9 : nesl_utility/PS-Simulink Converter  Commented=on  PhysicalDomain=network_engine_domain  SubClassName=ps_output  LeftPortType=input  RightPortType=output  PseudoPeriodic=off  Frequencies=[]  VectorFormat=inherit  Unit=inherit  AffineConversion=off
  Power Sensor : ee_lib/Sensors & Transducers/Power Sensor  measurement_type=1  averaging_period=1e-4 s
  Power Sensor1 : ee_lib/Sensors & Transducers/Power Sensor  measurement_type=1  averaging_period=1e-4 s
  Product1 : Product  Commented=on
  Reference Temp : fl_lib/Thermal/Thermal Sources/Temperature Source  temperature=0 degC
  Reference Temp1 : fl_lib/Thermal/Thermal Sources/Temperature Source  temperature=0 degC
  Reference Temp2 : fl_lib/Thermal/Thermal Sources/Temperature Source  temperature=0 degC
  ReferenceTemp3 : fl_lib/Thermal/Thermal Sources/Temperature Source  temperature=0 degC
  SOC : Scope
  SOC Calculation : Subsystem
  Scope : Scope
  Scope2 : Scope
  Simulink-PS Converter : nesl_utility/Simulink-PS Converter  PhysicalDomain=network_engine_domain  SubClassName=ps_input  LeftPortType=input  RightPortType=output  PseudoPeriodic=off  Frequencies=[]  NoiseDistribution=none  NoiseParameters=[]  Unit=1  AffineConversion=off  FilteringAndDerivatives=provide  SimscapeFilterOrder=1  InputFilterTimeConstant=0.001  UdotUserProvided=0
  Simulink-PS Converter2 : nesl_utility/Simulink-PS Converter  Commented=on  PhysicalDomain=network_engine_domain  SubClassName=ps_input  LeftPortType=input  RightPortType=output  PseudoPeriodic=off  Frequencies=[]  NoiseDistribution=none  NoiseParameters=[]  Unit=K/W  AffineConversion=off  FilteringAndDerivatives=provide  SimscapeFilterOrder=1  InputFilterTimeConstant=0.001  UdotUserProvided=0
  Simulink-PS Converter3 : nesl_utility/Simulink-PS Converter  PhysicalDomain=network_engine_domain  SubClassName=ps_input  LeftPortType=input  RightPortType=output  PseudoPeriodic=off  Frequencies=[]  NoiseDistribution=none  NoiseParameters=[]  Unit=K  AffineConversion=off  FilteringAndDerivatives=provide  SimscapeFilterOrder=1  InputFilterTimeConstant=0.001  UdotUserProvided=0
  Solver : nesl_utility/Solver Configuration  Commented=on  PhysicalDomain=network_engine_domain  SubClassName=solver  LeftPortType=input  RightPortType=generic  Tones=[]  Harmonics=[]  SimulateNoise=off  Profile=off  UseLocalSampling=off  EnableSwitchedLinearOptims=on  FrequencyDomain=off  UseCCode=off  RelTol=0.001  AbsTol=1e-06  MinStep=1e-09  ToWorkspace=off  RevertToSquareIcSolve=off  NumHomotopyIterations=100  PhasorMode=off  PhasorModeNumHarmonics=1  ConsistencySolver=NEWTON_FTOL  IndexReductionMethod=DerivativeReplacement  DoDC=off  ResidualTolerance=1e-09  ConsistencyTolSource=GLOBAL  ConsistencyAbsTol=0.001  ConsistencyRelTol=0.001  ConsistencyTolFactor=0.001  UseLocalSolver=off  LocalSolverChoice=NE_BACKWARD_EULER_ADVANCER  ResolveIndetEquations=on  FunctionEvalNumThread=1  LocalSolverSampleTime=0.001  DoFixedCost=off  MaxNonlinIter=3  MaxModeIter=2  ComputeImpulses=off  ImpulseIterations=2  LinearAlgebra=auto  LinearAlgebraNumThread=0  EquationFormulation=NE_TIME_EF  DelaysMemoryBudget=1024  AutomaticFiltering=on  FilteringTimeConstant=0.001  PartitionStorageMethod=AS_NEEDED  PartitionMemoryBudget=1024  PartitionMethod=ROBUST
  Tab Resistance : fl_lib/Electrical/Electrical Elements/Resistor  R=tabResis Ohm  i_specify=off  i_priority=None  i=0 A  i_nominal_specify=off  i_nominal_unit=A  i_nominal_value=1  v_specify=off  v_priority=None  v=0 V  v_nominal_specify=off  v_nominal_unit=V  v_nominal_value=1  mask(Resistor){}
  Thermal Reference3 : fl_lib/Thermal/Thermal Elements/Thermal Reference
  Thermal Reference4 : fl_lib/Thermal/Thermal Elements/Thermal Reference
  Thermal Resistance : fl_lib/Thermal/Thermal Elements/Thermal Resistance  resistance=thermistorContactRes K/W  T_specify=off  T_priority=None  T=0 K  T_nominal_specify=off  T_nominal_unit=K  T_nominal_value=1  Q_specify=off  Q_priority=None  Q=0 W  Q_nominal_specify=off  Q_nominal_unit=W  Q_nominal_value=1
  Total Heat Generated Scope : Scope
  Variable Resistor : fl_lib/Electrical/Electrical Elements/Variable Resistor  Rmin=0 Ohm  i_specify=off  i_priority=None  i=0 A  i_nominal_specify=off  i_nominal_unit=A  i_nominal_value=1  v_specify=off  v_priority=None  v=0 V  v_nominal_specify=off  v_nominal_unit=V  v_nominal_value=1
  Variable Thermal Resistance : fl_lib/Thermal/Thermal Elements/Variable Thermal Resistance  Commented=on  R_min=0 K/W  T_specify=off  T_priority=None  T=0 K  T_nominal_specify=off  T_nominal_unit=K  T_nominal_value=1  Q_specify=off  Q_priority=None  Q=0 W  Q_nominal_specify=off  Q_nominal_unit=W  Q_nominal_value=1
      settings: InternalSimscapePortConfiguration="{\"Bottom\":[],\"Left\":[{\"id\":\"A\",\"label\":\"A\",\"type\":\"foundation.thermal.thermal\"},{\"id\":\"R\",\"label\":\"R\",\"type\":\"input\"}],\"Right\":[{\"id\":\"B\",\"label\":\"B\",\"type\":\"foundation.thermal.thermal\"}],\"Top\":[]}"
  dOCVdT vs SOC : fl_lib/Physical Signals/Lookup Tables/PS Lookup Table (1D)  x=SOC  f=dOCVdT V/K  interp_method=simscape.enum.interpolation.linear  extrap_method=simscape.enum.extrapolation.nearest
  segment to container resistance : fl_lib/Thermal/Thermal Elements/Thermal Resistance  resistance=R_cb K/W  T_specify=off  T_priority=None  T=0 K  T_nominal_specify=off  T_nominal_unit=K  T_nominal_value=1  Q_specify=off  Q_priority=None  Q=0 W  Q_nominal_specify=off  Q_nominal_unit=W  Q_nominal_value=1
  segment to cover resistance : fl_lib/Thermal/Thermal Elements/Thermal Resistance  resistance=R_cb K/W  T_specify=off  T_priority=None  T=0 K  T_nominal_specify=off  T_nominal_unit=K  T_nominal_value=1  Q_specify=off  Q_priority=None  Q=0 W  Q_nominal_specify=off  Q_nominal_unit=W  Q_nominal_value=1
  Conn1 : PMIOPort  Side=Left
  Conn2 : PMIOPort  Port=2  Side=Right
  Conn3 : PMIOPort  Port=3  Side=Right
  Conn4 : PMIOPort  Port=4  Side=Right
  Conn5 : PMIOPort  Port=5  Side=Right
  wires:
  PS-Simulink Converter9/1 -> Gain2/1, Math Function/1
  Constant1/1 -> Product1/1
  SOC Calculation/1(SOC [0,1]) -> Simulink-PS Converter/1, SOC/1  "State of Charge [0,1]"
  Math Function/1 -> Gain1/1
  Gain2/1 -> Add/2
  Add/1 -> Product1/2
  Gain1/1 -> Add/1
  C to K conversion/1 -> Simulink-PS Converter3/1
  Integrator3/1 -> Total Heat Generated Scope/1
  PS-Simulink Converter3/1 -> SOC Calculation/1(I [A])
  PS-Simulink Converter16/1 -> Scope2/1
  Product1/1 -> Math Function1/1
  PS-Simulink Converter12/1 -> Entropic Negative Heat Generation/1
  PS-Simulink Converter15/1 -> Scope/1
  Constant/1 -> Add/3
  PS-Simulink Converter14/1 -> Integrator3/1
  Math Function1/1 -> Simulink-PS Converter2/1
  connections:
  Electrical Reference1/LConn1 -- Power Sensor1/LConn3 -- Tab Resistance/RConn1 -- Controlled Current Source1/RConn2
  Simulink-PS Converter2/RConn1 -- Variable Thermal Resistance/LConn2
  Cell Tab Resistance/LConn1 -- Cell tab/LConn1 -- Convective Heat Transfer1/LConn1 -- Thermal Resistance/LConn1 -- Interconnect Tab/LConn1 -- Heat Flow Rate Sensor3/RConn2
  Reference Temp1/LConn1 -- Cover Temp Sensor/RConn1
  Ambient Air/LConn1 -- Variable Thermal Resistance/RConn1
  Interconnect Resistance/LConn1 -- Heat Flow Rate Sensor3/LConn1
  IR vs Temperature Lookup/RConn1 -- Variable Resistor/LConn1
  PS Counter/RConn1 -- Motor Speed/LConn1
  Heat Flow Rate Sensor3/RConn1 -- PS Add/LConn2
  Controlled Current Source1/RConn1 -- PS Product2/LConn1 -- PS-Simulink Converter3/LConn1 -- Controlled Current Source/RConn1 -- Current Lookup/RConn1 -- PS-Simulink Converter16/LConn1
  Container Temp Sensor/LConn1 -- segment to container resistance/RConn1 -- Container/LConn1 -- Variable Thermal Resistance/LConn1
  Cell Temp (K)/LConn2 -- Conn3/RConn1 -- Cell Temperature Sensor/RConn2 -- IR vs Temperature Lookup/LConn1
  Variable Resistor/RConn1 -- Power Sensor/LConn3 -- Electrical Reference/LConn1 -- Controlled Current Source/RConn2
  Solver/RConn1 -- Motor Speed/RConn1 -- PS-Simulink Converter9/LConn1
  PS Counter1/RConn1 -- Current Lookup/LConn1
  Cell Internal Resistance/RConn2 -- Thermal Reference4/LConn1
  PS-Simulink Converter12/LConn1 -- PS Subtract/LConn2 -- PS Product2/RConn1
  Cell Tab Resistance/RConn1 -- segment to cover resistance/LConn1 -- segment to container resistance/LConn1 -- Cell Temperature Sensor/LConn1 -- " Fin1"/LConn1 -- "Cell "/LConn1 -- Heat Flow Rate Sensor4/RConn2
  Cover/LConn1 -- Conn1/RConn1 -- Cover Temp Sensor/LConn1 -- segment to cover resistance/RConn1
  dOCVdT vs SOC/RConn1 -- PS Product1/LConn1
  Interconnect Bolt/LConn1 -- Interconnect Nut/LConn1 -- Cell Tab Temp Sensor/LConn1 -- Thermal Resistance/RConn1
  Simulink-PS Converter/RConn1 -- dOCVdT vs SOC/LConn1
  Cell Internal Resistance/LConn1 -- Heat Flow Rate Sensor4/LConn1
  Reference Temp/LConn1 -- Container Temp Sensor/RConn1
  Power Sensor/LConn2 -- Variable Resistor/LConn2
  PS Product2/LConn2 -- PS Product1/RConn1
  Tab Resistance/LConn1 -- Power Sensor1/LConn2
  Controlled Current Source/LConn1 -- Power Sensor/LConn1
  PS Subtract/RConn1 -- Cell Internal Resistance/RConn1
  Heat Flow Rate Sensor5/RConn1 -- PS-Simulink Converter15/LConn1
  Cell Temp (K)/RConn1 -- PS Product1/LConn2
  Interconnect Resistance/RConn2 -- Thermal Reference3/LConn1
  PS-Simulink Converter14/LConn1 -- PS Add/RConn1
  ReferenceTemp3/LConn1 -- Cell Tab Temp Sensor/RConn1
  PS Subtract/LConn1 -- Power Sensor/RConn1
  Convective Heat Transfer1/RConn1 -- Heat Flow Rate Sensor5/LConn1
  Controlled Current Source1/LConn1 -- Power Sensor1/LConn1
  Heat Flow Rate Sensor5/RConn2 -- Ambient Air1/LConn1
  Cell Tab Temp Sensor/RConn2 -- Conn2/RConn1
  Cover Temp Sensor/RConn2 -- Conn4/RConn1
  Heat Flow Rate Sensor4/RConn1 -- PS Add/LConn1
  Cell Temp (K)/LConn1 -- Simulink-PS Converter3/RConn1
  Container Temp Sensor/RConn2 -- Conn5/RConn1
  Power Sensor1/RConn1 -- Interconnect Resistance/RConn1
  Cell Temperature Sensor/RConn1 -- Reference Temp2/LConn1

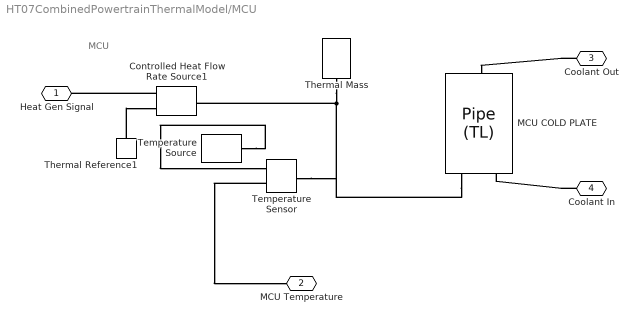
== system HT07CombinedPowertrainThermalModel/MCU ==
  note: MCU
  Controlled Heat Flow Rate Source1 : fl_lib/Thermal/Thermal Sources/Controlled Heat Flow Rate Source
  MCU COLD PLATE : SimscapeFluids_lib/Thermal Liquid/Pipes & Fittings/Pipe (TL)  dynamic_compressibility=simscape.enum.onoff.off  inertia=simscape.enum.onoff.off  num_segments=1  pipe_length=mcuColdPlateLength m  area=mcuColdPlateFlowArea m^2  wall_spec=fluids.thermal_liquid.pipes_fittings.enum.wall_spec.rigid  Dh=mcuColdPlateDiameter m  wall_compliance=1.2e-6 m/MPa  wall_time_constant=0.01 s  elevation_spec=foundation.enum.constant_variable.constant  elevation_gain=0 m  g=9.81 m/s^2  pressure_loss_spec=fluids.thermal_liquid.pipes_fittings.enum.PressureLossSpec.Nominal  local_pressure_loss_spec=fluids.thermal_liquid.pipes_fittings.enum.LocalLossSpec.AggregateLength  length_add=0 m  loss_coefficient=0.1  roughness=tubeRoughness m  Re_friction_TLU=[400, 1000, 1500, 3000, 4000, 6000, 10000, 20000, 40000, 60000, 100000, 100000000]  friction_factor_TLU=[.264, .112, .071, .0417, .0387, .0268, .025, .0232, .0226, .022, .0214, .0214]  shape_factor=64  Re_lam=2000  Re_tur=4000  mdot_nominal=12 kg/min  p_diff_nominal=0.3 bar  mdot_threshold=1e-6 kg/s  heat_transfer_spec=fluids.thermal_liquid.pipes_fittings.enum.HeatTransferSpec.DittusBoelter  mdot_nominal_heat=[.1, 1] kg/s  T_in_nominal=[293.15, 293.15] K  T_out_nominal=[300, 300] K  p_in_nominal_heat=[.101325, .101325] MPa  T_wall_nominal=[303.15, 303.15] K  a_coeff=0.023  b_Re_power=0.8  c_Pr_power=0.4  Nu_lam=3.66  Re_Colburn_TLU=[100, 150, 1000]  Colburn_factor_TLU=[.019, .013, .002]  Re_Nu_TLU=[100, 150, 1000]  Pr_Nu_TLU=[1, 10]  Nu_TLU=[3.72, 4.21; 3.75, 4.44; 4.21, 7.15]  T0_vec=Tamb degC  p0_vec=0.101325 MPa  mdot0=0.1 kg/s
  Temperature Sensor : fl_lib/Thermal/Thermal Sensors/Temperature Sensor
  Temperature Source : fl_lib/Thermal/Thermal Sources/Temperature Source  temperature=0 degC
  Thermal Mass : fl_lib/Thermal/Thermal Elements/Thermal Mass  mass=coldPlateMassMCU kg  sp_heat=cAl J/(K*kg)  num_ports=foundation.enum.numPorts2.one  T_specify=on  T_priority=High  T=Tamb degC  T_nominal_specify=off  T_nominal_unit=K  T_nominal_value=1  Q_specify=off  Q_priority=None  Q=0 W  Q_nominal_specify=off  Q_nominal_unit=W  Q_nominal_value=1
  Thermal Reference1 : fl_lib/Thermal/Thermal Elements/Thermal Reference
  Heat Gen Signal : PMIOPort  Side=Left
  MCU Temperature : PMIOPort  Port=2  Side=Left
  Coolant Out : PMIOPort  Port=3  Side=Right
  Coolant In : PMIOPort  Port=4  Side=Right
  connections:
  Temperature Sensor/RConn2 -- MCU Temperature/RConn1
  MCU COLD PLATE/LConn2 -- Temperature Sensor/LConn1 -- Controlled Heat Flow Rate Source1/LConn1 -- Thermal Mass/LConn1
  Temperature Source/LConn1 -- Temperature Sensor/RConn1
  Thermal Reference1/LConn1 -- Controlled Heat Flow Rate Source1/RConn2
  Coolant In/RConn1 -- MCU COLD PLATE/LConn1
  Coolant Out/RConn1 -- MCU COLD PLATE/RConn1
  Controlled Heat Flow Rate Source1/RConn1 -- Heat Gen Signal/RConn1

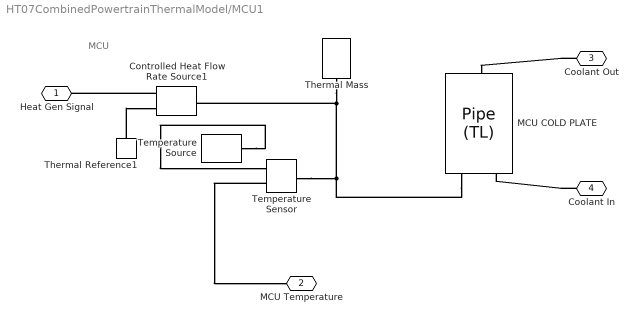
== system HT07CombinedPowertrainThermalModel/MCU1 ==
  note: MCU
  Controlled Heat Flow Rate Source1 : fl_lib/Thermal/Thermal Sources/Controlled Heat Flow Rate Source
  MCU COLD PLATE : SimscapeFluids_lib/Thermal Liquid/Pipes & Fittings/Pipe (TL)  dynamic_compressibility=simscape.enum.onoff.off  inertia=simscape.enum.onoff.off  num_segments=1  pipe_length=mcuColdPlateLength m  area=mcuColdPlateFlowArea m^2  wall_spec=fluids.thermal_liquid.pipes_fittings.enum.wall_spec.rigid  Dh=mcuColdPlateDiameter m  wall_compliance=1.2e-6 m/MPa  wall_time_constant=0.01 s  elevation_spec=foundation.enum.constant_variable.constant  elevation_gain=0 m  g=9.81 m/s^2  pressure_loss_spec=fluids.thermal_liquid.pipes_fittings.enum.PressureLossSpec.Nominal  local_pressure_loss_spec=fluids.thermal_liquid.pipes_fittings.enum.LocalLossSpec.AggregateLength  length_add=0 m  loss_coefficient=0.1  roughness=tubeRoughness m  Re_friction_TLU=[400, 1000, 1500, 3000, 4000, 6000, 10000, 20000, 40000, 60000, 100000, 100000000]  friction_factor_TLU=[.264, .112, .071, .0417, .0387, .0268, .025, .0232, .0226, .022, .0214, .0214]  shape_factor=64  Re_lam=2000  Re_tur=4000  mdot_nominal=12 kg/min  p_diff_nominal=0.3 bar  mdot_threshold=1e-6 kg/s  heat_transfer_spec=fluids.thermal_liquid.pipes_fittings.enum.HeatTransferSpec.DittusBoelter  mdot_nominal_heat=[.1, 1] kg/s  T_in_nominal=[293.15, 293.15] K  T_out_nominal=[300, 300] K  p_in_nominal_heat=[.101325, .101325] MPa  T_wall_nominal=[303.15, 303.15] K  a_coeff=0.023  b_Re_power=0.8  c_Pr_power=0.4  Nu_lam=3.66  Re_Colburn_TLU=[100, 150, 1000]  Colburn_factor_TLU=[.019, .013, .002]  Re_Nu_TLU=[100, 150, 1000]  Pr_Nu_TLU=[1, 10]  Nu_TLU=[3.72, 4.21; 3.75, 4.44; 4.21, 7.15]  T0_vec=Tamb degC  p0_vec=0.101325 MPa  mdot0=0.1 kg/s
  Temperature Sensor : fl_lib/Thermal/Thermal Sensors/Temperature Sensor
  Temperature Source : fl_lib/Thermal/Thermal Sources/Temperature Source  temperature=0 degC
  Thermal Mass : fl_lib/Thermal/Thermal Elements/Thermal Mass  mass=coldPlateMassMCU kg  sp_heat=cAl J/(K*kg)  num_ports=foundation.enum.numPorts2.one  T_specify=on  T_priority=High  T=Tamb degC  T_nominal_specify=off  T_nominal_unit=K  T_nominal_value=1  Q_specify=off  Q_priority=None  Q=0 W  Q_nominal_specify=off  Q_nominal_unit=W  Q_nominal_value=1
  Thermal Reference1 : fl_lib/Thermal/Thermal Elements/Thermal Reference
  Heat Gen Signal : PMIOPort  Side=Left
  MCU Temperature : PMIOPort  Port=2  Side=Left
  Coolant Out : PMIOPort  Port=3  Side=Right
  Coolant In : PMIOPort  Port=4  Side=Right
  connections:
  Temperature Sensor/RConn2 -- MCU Temperature/RConn1
  MCU COLD PLATE/LConn2 -- Temperature Sensor/LConn1 -- Thermal Mass/LConn1 -- Controlled Heat Flow Rate Source1/LConn1
  Temperature Source/LConn1 -- Temperature Sensor/RConn1
  Thermal Reference1/LConn1 -- Controlled Heat Flow Rate Source1/RConn2
  Coolant In/RConn1 -- MCU COLD PLATE/LConn1
  Coolant Out/RConn1 -- MCU COLD PLATE/RConn1
  Controlled Heat Flow Rate Source1/RConn1 -- Heat Gen Signal/RConn1
